simulink model "sampleModel1731"  (R2023a)
settings: Solver=VariableStepAuto  StartTime=0.0  StopTime=10.0  RelTol=1e-3
libraries: simulink x2, hdlsllib x2
settings Model: Creator=user1  LastModifiedBy=user1

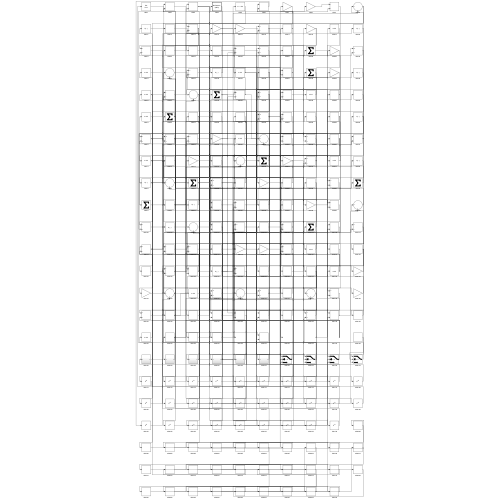
[thumbnail: Simulink's stored preview of the top-level diagram]
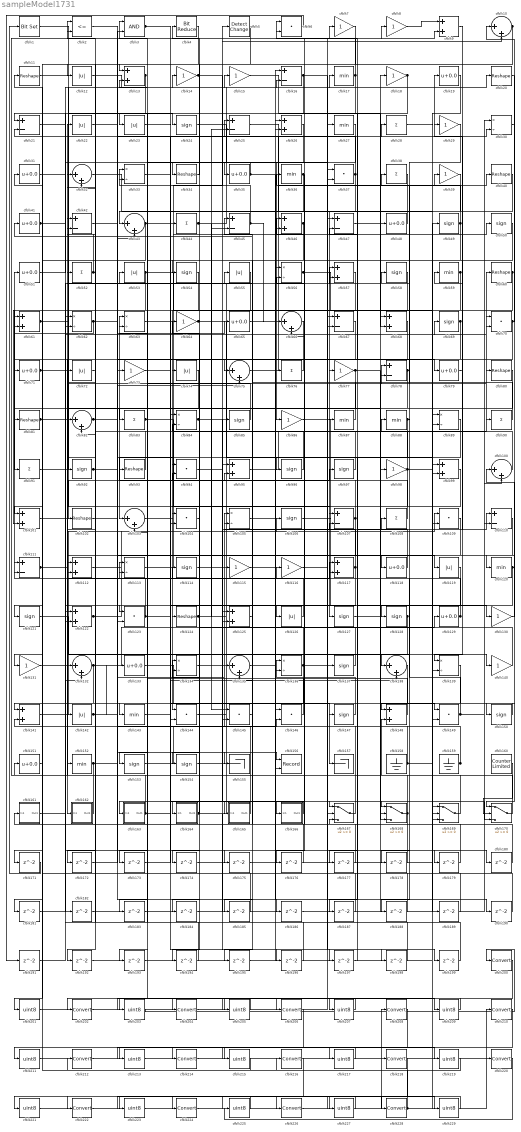
== system sampleModel1731 ==
  cfblk1 : simulink/Logic and Bit Operations/Bit Set  iBit=0
      settings: LibrarySourceBlock=|
      | hdlsllib/Logic and Bit
      | Operations/Bit Set
  cfblk{10,32,43,66,75,82,100,103,132,135,138} (11 alike) : Sum  Inputs=|++
  cfblk{9,13,26,46,57,61,68,95,99,101,112,117,122,125,141,148} (16 alike) : Sum
  cfblk{11,20,34,40,60,80..81,93,102,124} (10 alike) : Reshape
  cfblk{6,37,70,94,104,109,123,144..146,149} (11 alike) : DotProduct  OutDataTypeStr=Inherit: Inherit via internal rule
  cfblk{30,33,56,62..63,84,89,105,113,134,136,139} (12 alike) : Product  Inputs=*/  RndMeth=Zero  SaturateOnIntegerOverflow=on
  cfblk{24,49..50,54,58,69,85,92,96..97,106,114,121,127..128,137,147,150,153..154} (20 alike) : Signum
  cfblk{16,21,25,42,45,47,67,78,107,110..111} (11 alike) : Sum  Inputs=+-
  cfblk{28,38,44,52,76,83,90..91,108} (9 alike) : Sum  Inputs=+
  cfblk{7..8,14..15,18,29,39,64,73,77,86,98,115..116,130..131,140} (17 alike) : Gain
  cfblk{19,31,35,41,48,51,65,71,79,118,129,133,151} (13 alike) : Bias  Bias=0.0  SaturateOnIntegerOverflow=off
  cfblk{12,22..23,53,55,72,74,119,126,142} (10 alike) : Abs  SaturateOnIntegerOverflow=off
  cfblk{17,27,36,59,87..88,120,143,152} (9 alike) : MinMax
  cfblk155 : Terminator
  cfblk156 : Record  FileSettingsInternal="{\"entries\":[{\"content\":{\"excelSettings\":{\"content\":{},\"type\":\"Streamout.ExcelSettings\"}},\"type\":\"Streamout.FileSettingStorage\",\"uuid\":\"\"}],\"packageUris\":[\"http:\\/\\/schema.mathworks.com\\/mf0\\/streamout_blocks\\/R2020a\"],\"version\":\"1.0\"}"  Layout=[1 1]  SignalsInternal="{\"entries\":[{\"content\":{\"signals\":[{\"content\":{\"blockPath\":[],\"dimensions\":[1],\"domain\":\"\",\"lineColor\":\"#a2142f\",\"plots\":[1],\"port\":1,\"signalID\":3459,\"signalName\":\"XY Graph:1\"},\"type\":\"RecordBlkView.Signal\",\"uuid\":\"\"},{\"content\":{\"blockPath\":[],\"dimensions\":[1],\"domain\":\"\",\"lineColor\":\"#139fff\",\"plots\":[1],\"port\":2,\"signalID\":3462,\"signalName\":\"XY Graph:2\"},\"type\":\"RecordBlkView.Signal\",\"uuid\":\"\"}]},\"type\":\"RecordBlkView.InputSignals\",\"uuid\":\"\"}],\"packageUris\":[\"http:\\/\\/schema.mathworks.com\\/mf0\\/streamout_blocks\\/R2020a\"],\"version\":\"1.0\"}"  VisualizationBindings="{\"xyplotplugin\":{\"info\":[{\"series\":[{\"bindingParametersList\":[{\"parameter\":\"X-Axis\",\"signalID\":3459,\"signalName\":\"XY Graph:1\"},{\"parameter\":\"Y-Axis\",\"signalID\":3462,\"signalName\":\"XY Graph:2\"}],\"seriesID\":62333}],\"subplotID\":1}]}}"  CompatibilityTag=XY  st=-1
  cfblk157 : Terminator
  cfblk158 : Ground
  cfblk159 : Ground
  cfblk160 : hdlsllib/Sources/Counter Limited  uplimit=7  tsamp=-1
  cfblk161 : Subsystem
      settings: LibrarySourceBlock=|
      | hdlsllib/Ports &
      | Subsystems/Subsystem
  cfblk162 : Subsystem
      settings: LibrarySourceBlock=|
      | hdlsllib/Ports &
      | Subsystems/Subsystem
  cfblk163 : Subsystem
      settings: LibrarySourceBlock=|
      | hdlsllib/Ports &
      | Subsystems/Subsystem
  cfblk164 : Subsystem
      settings: LibrarySourceBlock=|
      | hdlsllib/Ports &
      | Subsystems/Subsystem
  cfblk165 : Subsystem
      settings: LibrarySourceBlock=|
      | hdlsllib/Ports &
      | Subsystems/Subsystem
  cfblk166 : Subsystem
      settings: LibrarySourceBlock=|
      | hdlsllib/Ports &
      | Subsystems/Subsystem
  cfblk{167..170} (4 alike) : Switch  SaturateOnIntegerOverflow=off  InputSameDT=off
  cfblk{171..199} (29 alike) : Delay  SampleTime=1
  cfblk2 : RelationalOperator  Operator=<=  OutDataTypeStr=boolean  InputSameDT=off
  cfblk{200,202,204,206,208,210,212,214,216,218,220,222,224,226,228} (15 alike) : DataTypeConversion  SaturateOnIntegerOverflow=off  RndMeth=Floor
  cfblk{201,203,205,207,209,211,213,215,217,219,221,223,225,227,229} (15 alike) : DataTypeConversion  OutDataTypeStr=uint8  SaturateOnIntegerOverflow=off  RndMeth=Floor
  cfblk3 : Logic  AllPortsSameDT=off  OutDataTypeStr=boolean
  cfblk4 : hdlsllib/Logic and Bit Operations/Bit Reduce  mode=AND
  cfblk5 : simulink/Logic and Bit Operations/Detect Change  vinit=0  OutDataTypeStr=boolean
      settings: LibrarySourceBlock=|
      | hdlsllib/Logic and Bit
      | Operations/Detect
      | Change
  wires:
  cfblk68/1 -> cfblk144/1
  cfblk154/1 -> cfblk58/1
  cfblk54/1 -> cfblk124/1
  cfblk131/1 -> cfblk106/1
  cfblk108/1 -> cfblk63/1
  cfblk88/1 -> cfblk103/1, cfblk148/1
  cfblk165/1(Out1) -> cfblk105/1
  cfblk122/1 -> cfblk16/1, cfblk57/1
  cfblk48/1 -> cfblk43/1
  cfblk26/1 -> cfblk86/1
  cfblk152/1 -> cfblk8/1, cfblk146/2, cfblk135/1
  cfblk91/1 -> cfblk15/1
  cfblk5/1 -> cfblk13/1
  cfblk106/1 -> cfblk59/1
  cfblk41/1 -> cfblk180/1, cfblk181/1
  cfblk123/1 -> cfblk51/1, cfblk147/1
  cfblk113/1 -> cfblk50/1
  cfblk134/1 -> cfblk110/1
  cfblk65/1 -> cfblk40/1
  cfblk125/1 -> cfblk161/1(In1)
  cfblk75/1 -> cfblk19/1
  cfblk70/1 -> cfblk91/1, cfblk10/1
  cfblk124/1 -> cfblk76/1, cfblk107/2, cfblk25/2
  cfblk129/1 -> cfblk46/1, cfblk32/2
  cfblk30/1 -> cfblk150/1
  cfblk12/1 -> cfblk14/1
  cfblk11/1 -> cfblk83/1
  cfblk69/1 -> cfblk145/2, cfblk92/1, cfblk184/1
  cfblk86/1 -> cfblk128/1
  cfblk46/1 -> cfblk135/2, cfblk183/1
  cfblk95/1 -> cfblk88/1
  cfblk1/1 -> cfblk24/1
  cfblk52/1 -> cfblk22/1, cfblk82/2
  cfblk42/1 -> cfblk20/1
  cfblk146/1 -> cfblk134/1
  cfblk121/1 -> cfblk140/1
  cfblk14/1 -> cfblk119/1, cfblk10/2
  cfblk25/1 -> cfblk127/1
  cfblk43/1 -> cfblk131/1, cfblk168/2
  cfblk40/1 -> cfblk144/2
  cfblk38/1 -> cfblk123/1
  cfblk112/1 -> cfblk26/2
  cfblk44/1 -> cfblk17/1, cfblk145/1
  cfblk66/1 -> cfblk162/1(In1)
  cfblk7/1 -> cfblk12/1
  cfblk80/1 -> cfblk123/2
  cfblk9/1 -> cfblk139/1
  cfblk18/1 -> cfblk77/1, cfblk61/1
  cfblk79/1 -> cfblk29/1
  cfblk87/1 -> cfblk41/1
  cfblk8/1 -> cfblk9/1
  cfblk103/1 -> cfblk60/1
  cfblk141/1 -> cfblk117/1
  cfblk111/1 -> cfblk109/1, cfblk70/2
  cfblk85/1 -> cfblk33/1
  cfblk58/1 -> cfblk96/1
  cfblk83/1 -> cfblk107/1, cfblk80/1
  cfblk81/1 -> cfblk78/1, cfblk70/1
  cfblk164/1(Out1) -> cfblk108/1, cfblk114/1, cfblk197/1, cfblk198/1
  cfblk76/1 -> cfblk74/1
  cfblk35/1 -> cfblk34/1, cfblk99/2, cfblk190/1
  cfblk136/1 -> cfblk95/2, cfblk9/2, cfblk195/1
  cfblk132/1 -> cfblk47/1, cfblk171/1
  cfblk32/1 -> cfblk89/1
  cfblk101/1 -> cfblk97/1
  cfblk34/1 -> cfblk4/1
  cfblk17/1 -> cfblk153/1, cfblk6/2
  cfblk107/1 -> cfblk55/1, cfblk193/1
  cfblk166/1(Out1) -> cfblk163/1(In1)
  cfblk147/1 -> cfblk136/1
  cfblk144/1 -> cfblk129/1
  cfblk162/1(Out1) -> cfblk42/1
  cfblk13/1 -> cfblk21/1, cfblk23/1
  cfblk109/1 -> cfblk112/1
  cfblk100/1 -> cfblk2/1
  cfblk77/1 -> cfblk81/1, cfblk149/1
  cfblk92/1 -> cfblk73/1, cfblk94/1, cfblk75/2
  cfblk110/1 -> cfblk164/1(In1)
  cfblk150/1 -> cfblk141/1
  cfblk33/1 -> cfblk35/1
  cfblk36/1 -> cfblk46/2, cfblk166/1(In1)
  cfblk63/1 -> cfblk5/1
  cfblk47/1 -> cfblk48/1
  cfblk49/1 -> cfblk104/1, cfblk6/1
  cfblk114/1 -> cfblk30/1
  cfblk105/1 -> cfblk167/1
  cfblk4/1 -> cfblk142/1
  cfblk158/1 -> cfblk49/1, cfblk21/2
  cfblk84/1 -> cfblk18/1, cfblk170/3
  cfblk127/1 -> cfblk39/1
  cfblk10/1 -> cfblk101/1, cfblk54/1
  cfblk73/1 -> cfblk126/1
  cfblk3/1 -> cfblk130/1, cfblk138/2, cfblk175/1
  cfblk29/1 -> cfblk138/1
  cfblk64/1 -> cfblk169/1, cfblk45/2
  cfblk96/1 -> cfblk53/1
  cfblk135/1 -> cfblk69/1
  cfblk74/1 -> cfblk143/1
  cfblk137/1 -> cfblk64/1
  cfblk24/1 -> cfblk137/1
  cfblk37/1 -> cfblk136/2, cfblk11/1
  cfblk97/1 -> cfblk33/2
  cfblk153/1 -> cfblk85/1
  cfblk169/1 -> cfblk84/2
  cfblk57/1 -> cfblk104/2
  cfblk126/1 -> cfblk102/1
  cfblk142/1 -> cfblk28/1, cfblk133/1
  cfblk94/1 -> cfblk156/1
  cfblk45/1 -> cfblk3/1, cfblk66/1
  cfblk55/1 -> cfblk121/1
  cfblk148/1 -> cfblk93/1
  cfblk163/1(Out1) -> cfblk25/1, cfblk72/1
  cfblk149/1 -> cfblk116/1, cfblk100/2
  cfblk15/1 -> cfblk68/1
  cfblk78/1 -> cfblk132/1, cfblk38/1
  cfblk90/1 -> cfblk52/1
  cfblk120/1 -> cfblk170/1, cfblk177/1, cfblk178/1
  cfblk160/1 -> cfblk170/2
  cfblk21/1 -> cfblk37/2
  cfblk117/1 -> cfblk45/1, cfblk122/2
  cfblk133/1 -> cfblk157/1
  cfblk151/1 -> cfblk111/1
  cfblk140/1 -> cfblk36/1
  cfblk159/1 -> cfblk31/1, cfblk134/2, cfblk113/2, cfblk94/2
  cfblk22/1 -> cfblk3/2
  cfblk53/1 -> cfblk71/1, cfblk68/2
  cfblk71/1 -> cfblk115/1, cfblk168/3
  cfblk115/1 -> cfblk168/1
  cfblk39/1 -> cfblk156/2
  cfblk168/1 -> cfblk152/1, cfblk148/2, cfblk2/2, cfblk167/3
  cfblk118/1 -> cfblk7/1
  cfblk2/1 -> cfblk155/1
  cfblk143/1 -> cfblk44/1
  cfblk19/1 -> cfblk89/2
  cfblk50/1 -> cfblk139/2
  cfblk60/1 -> cfblk165/1(In1), cfblk101/2
  cfblk167/1 -> cfblk56/2
  cfblk128/1 -> cfblk154/1, cfblk172/1
  cfblk20/1 -> cfblk120/1
  cfblk170/1 -> cfblk113/1
  cfblk62/1 -> cfblk79/1, cfblk87/1, cfblk61/2
  cfblk56/1 -> cfblk99/1, cfblk30/2
  cfblk93/1 -> cfblk32/1
  cfblk31/1 -> cfblk82/1
  cfblk130/1 -> cfblk100/1
  cfblk16/1 -> cfblk62/2, cfblk179/1
  cfblk59/1 -> cfblk67/2, cfblk75/1
  cfblk61/1 -> cfblk98/1, cfblk57/2
  cfblk51/1 -> cfblk16/2
  cfblk98/1 -> cfblk125/2, cfblk90/1, cfblk42/2
  cfblk82/1 -> cfblk65/1, cfblk118/1
  cfblk171/1 -> cfblk1/1
  cfblk172/1 -> cfblk43/2
  cfblk139/1 -> cfblk173/1
  cfblk173/1 -> cfblk84/1
  cfblk99/1 -> cfblk174/1
  cfblk174/1 -> cfblk56/1
  cfblk175/1 -> cfblk109/2
  cfblk138/1 -> cfblk176/1
  cfblk176/1 -> cfblk103/2
  cfblk177/1 -> cfblk167/2
  cfblk178/1 -> cfblk66/2
  cfblk179/1 -> cfblk105/2
  cfblk180/1 -> cfblk26/1
  cfblk181/1 -> cfblk132/2
  cfblk161/1(Out1) -> cfblk182/1
  cfblk182/1 -> cfblk125/1
  cfblk183/1 -> cfblk37/1
  cfblk184/1 -> cfblk110/2
  cfblk145/1 -> cfblk185/1
  cfblk185/1 -> cfblk63/2
  cfblk102/1 -> cfblk186/1
  cfblk186/1 -> cfblk78/2
  cfblk89/1 -> cfblk187/1
  cfblk187/1 -> cfblk95/1
  cfblk119/1 -> cfblk188/1
  cfblk188/1 -> cfblk141/2
  cfblk28/1 -> cfblk189/1
  cfblk189/1 -> cfblk111/2
  cfblk190/1 -> cfblk117/2
  cfblk6/1 -> cfblk191/1
  cfblk191/1 -> cfblk62/1
  cfblk72/1 -> cfblk192/1
  cfblk192/1 -> cfblk169/2
  cfblk193/1 -> cfblk169/3
  cfblk104/1 -> cfblk194/1
  cfblk194/1 -> cfblk122/1
  cfblk195/1 -> cfblk146/1
  cfblk23/1 -> cfblk196/1
  cfblk196/1 -> cfblk13/2
  cfblk197/1 -> cfblk47/2
  cfblk198/1 -> cfblk112/2
  cfblk116/1 -> cfblk199/1
  cfblk199/1 -> cfblk67/1
  cfblk67/1 -> cfblk201/1
  cfblk201/1 -> cfblk27/1
  cfblk27/1 -> cfblk203/1
  cfblk203/1 -> cfblk200/1
  cfblk200/1 -> cfblk205/1
  cfblk205/1 -> cfblk202/1
  cfblk202/1 -> cfblk207/1
  cfblk207/1 -> cfblk204/1
  cfblk204/1 -> cfblk209/1
  cfblk209/1 -> cfblk206/1
  cfblk206/1 -> cfblk211/1
  cfblk211/1 -> cfblk208/1
  cfblk208/1 -> cfblk213/1
  cfblk213/1 -> cfblk210/1
  cfblk210/1 -> cfblk215/1
  cfblk215/1 -> cfblk212/1
  cfblk212/1 -> cfblk217/1
  cfblk217/1 -> cfblk214/1
  cfblk214/1 -> cfblk219/1
  cfblk219/1 -> cfblk216/1
  cfblk216/1 -> cfblk221/1
  cfblk221/1 -> cfblk218/1
  cfblk218/1 -> cfblk223/1
  cfblk223/1 -> cfblk220/1
  cfblk220/1 -> cfblk225/1
  cfblk225/1 -> cfblk222/1
  cfblk226/1 -> cfblk228/1
  cfblk222/1 -> cfblk227/1
  cfblk227/1 -> cfblk224/1
  cfblk228/1 -> cfblk149/2, cfblk151/1
  cfblk224/1 -> cfblk229/1
  cfblk229/1 -> cfblk226/1

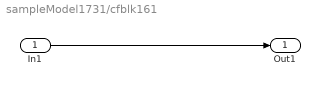
== system sampleModel1731/cfblk161 ==
  In1 : Inport
  Out1 : Outport
  wires:
  In1/1 -> Out1/1

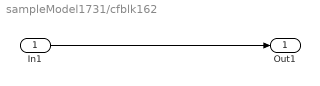
== system sampleModel1731/cfblk162 ==
  In1 : Inport
  Out1 : Outport
  wires:
  In1/1 -> Out1/1

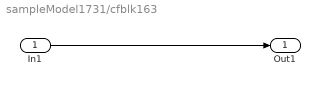
== system sampleModel1731/cfblk163 ==
  In1 : Inport
  Out1 : Outport
  wires:
  In1/1 -> Out1/1

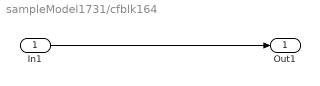
== system sampleModel1731/cfblk164 ==
  In1 : Inport
  Out1 : Outport
  wires:
  In1/1 -> Out1/1

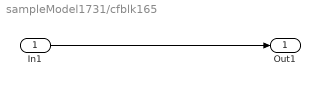
== system sampleModel1731/cfblk165 ==
  In1 : Inport
  Out1 : Outport
  wires:
  In1/1 -> Out1/1

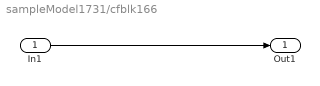
== system sampleModel1731/cfblk166 ==
  In1 : Inport
  Out1 : Outport
  wires:
  In1/1 -> Out1/1
